simulink model "PID_new_1"  (R2015a)
settings: Solver=ode45  StartTime=0.0  StopTime=2  RelTol=1e-3
libraries: simulink_extras x1, simulink x1, powerlib_meascontrol x1
settings Model: Creator=Pranabendra  LastModifiedBy=Pranabendra

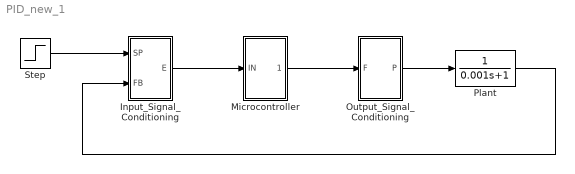
== system PID_new_1 ==
  Input_Signal_Conditioning : Subsystem
  Microcontroller : Subsystem
  Output_Signal_Conditioning : Subsystem
  Plant : TransferFcn  Denominator=[0.001 1]
  Step : Step  After=5  SampleTime=0
  wires:
  Step/1 -> Input_Signal_Conditioning/1(SP)
  Input_Signal_Conditioning/1(E) -> Microcontroller/1(IN)
  Microcontroller/1(OUT) -> Output_Signal_Conditioning/1(F)
  Output_Signal_Conditioning/1(P) -> Plant/1
  Plant/1 -> Input_Signal_Conditioning/2(FB)

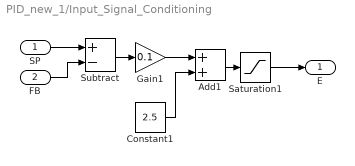
== system PID_new_1/Input_Signal_Conditioning ==
  SP : Inport
  FB : Inport  Port=2
  Add1 : Sum
  Constant1 : Constant  Value=2.5
  Gain1 : Gain  Gain=0.1
  Saturation1 : Saturate  UpperLimit=4.95  LowerLimit=0.05
  Subtract : Sum  Inputs=+-
  E : Outport
  wires:
  Constant1/1 -> Add1/2
  Add1/1 -> Saturation1/1
  SP/1 -> Subtract/1
  Subtract/1 -> Gain1/1
  Gain1/1 -> Add1/1
  Saturation1/1 -> E/1
  FB/1 -> Subtract/2

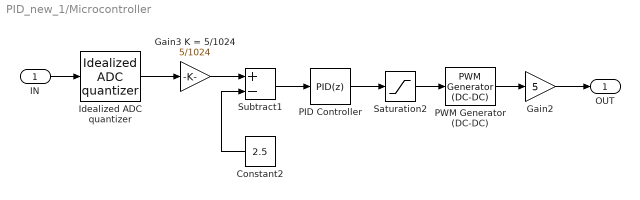
== system PID_new_1/Microcontroller ==
  IN : Inport
  Constant2 : Constant  Value=2.5
  Gain2 : Gain  Gain=5
  Gain3 K = 5/1024 : Gain  Gain=5/1024
  Idealized ADC quantizer : simulink_extras/Additional Discrete/Idealized ADC quantizer  NumberOfConverterBits=10  Vmin=0  Vmax=5  OutputDataType=int16  OutputNegativeValues=off
  PID Controller : simulink/Continuous/PID Controller  Controller=PID  TimeDomain=Discrete-time  SampleTime=0.0002  IntegratorMethod=Forward Euler  FilterMethod=Forward Euler  Form=Parallel  UseFilter=on  ControllerParametersSource=internal  P=0.004  I=20  D=0  N=100  InitialConditionSource=internal  InitialConditionForIntegrator=0  InitialConditionForFilter=0  ExternalReset=none  LimitOutput=off  UpperSaturationLimit=inf  LowerSaturationLimit=-inf  LinearizeAsGain=on  AntiWindupMode=none  Kb=1  TrackingMode=off  Kt=1  PParamMin=[]  PParamMax=[]  IParamMin=[]  IParamMax=[]  DParamMin=[]  DParamMax=[]  NParamMin=[]  NParamMax=[]  KbParamMin=[]  KbParamMax=[]  KtParamMin=[]  KtParamMax=[]  POutMin=[]  POutMax=[]  IOutMin=[]  IOutMax=[]  DOutMin=[]  DOutMax=[]  NOutMin=[]  NOutMax=[]  KbOutMin=[]  KbOutMax=[]  KtOutMin=[]  KtOutMax=[]  IntegratorOutMin=[]  IntegratorOutMax=[]  FilterOutMin=[]  FilterOutMax=[]  SumOutMin=[]  SumOutMax=[]  SumI1OutMin=[]  SumI1OutMax=[]  SumI2OutMin=[]  SumI2OutMax=[]  SumI3OutMin=[]  SumI3OutMax=[]  SumDOutMin=[]  SumDOutMax=[]  SaturationOutMin=[]  SaturationOutMax=[]  IntegratorContinuousStateAttributes=''  IntegratorStateMustResolveToSignalObject=off  IntegratorRTWStateStorageClass=Auto  FilterContinuousStateAttributes=''  FilterStateMustResolveToSignalObject=off  FilterRTWStateStorageClass=Auto  DifferentiatorICPrevScaledInput=0  DifferentiatorOutMin=[]  DifferentiatorOutMax=[]
  PWM Generator (DC-DC) : powerlib_meascontrol/Pulse & Signal Generators/PWM Generator (DC-DC)  Fsw=100000  Ts=0
  Saturation2 : Saturate  UpperLimit=0.995  LowerLimit=0.005
  Subtract1 : Sum  Inputs=+-
  OUT : Outport
  wires:
  PWM Generator (DC-DC)/1 -> Gain2/1
  Gain2/1 -> OUT/1
  PID Controller/1 -> Saturation2/1
  Saturation2/1 -> PWM Generator (DC-DC)/1
  Subtract1/1 -> PID Controller/1
  Constant2/1 -> Subtract1/2
  IN/1 -> Idealized ADC quantizer/1
  Gain3 K = 5/1024/1 -> Subtract1/1
  Idealized ADC quantizer/1 -> Gain3 K = 5/1024/1

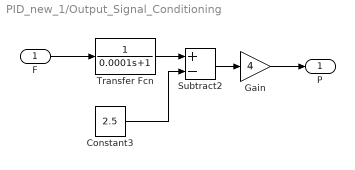
== system PID_new_1/Output_Signal_Conditioning ==
  F : Inport
  "Constant3 " : Constant  Value=2.5
  Gain : Gain  Gain=4
  Subtract2 : Sum  Inputs=+-
  Transfer Fcn : TransferFcn  Denominator=[0.0001 1]
  P : Outport
  wires:
  Transfer Fcn/1 -> Subtract2/1
  "Constant3 "/1 -> Subtract2/2
  Gain/1 -> P/1
  Subtract2/1 -> Gain/1
  F/1 -> Transfer Fcn/1
